simulink model "test_model_desktop_realtime"  (R2020b)
settings: Solver=FixedStepDiscrete  StartTime=0.0  StopTime=2  FixedStep=Ts  RelTol=1e-3
libraries: sldrtlib x1, simulink x1
settings Model: SimulationMode=external  ExtModeTrigDuration=100000  Creator=umbe  LastModifiedBy=irong
settings RTWCC: Description=Simulink Desktop Real-Time  SystemTargetFile=sldrt.tlc  TemplateMakefile=sldrt.tmf  RTWCompilerOptimization=on
settings CodeAppCC: MaxIdLength=95
settings SimulinkDesktopRealTimeCC: TargetPreCompLibLocation=D:\MATLAB\R2020b\toolbox\sldrt\lib\win64

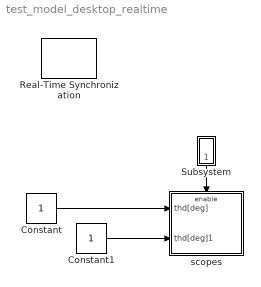
== system test_model_desktop_realtime ==
  Constant : Constant
  Constant1 : Constant
  Real-Time Synchronization : sldrtlib/Real-Time Synchronization  SampleTime=0.1  MaxMissedTicks=10  ShowMissedTicks=off  YieldWhenWaiting=off
  Subsystem : Subsystem
  scopes : Subsystem
  wires:
  Subsystem/1(1.0 s) -> scopes/Enable
  Constant/1 -> scopes/1(thd[deg])
  Constant1/1 -> scopes/2(thd[deg]1)

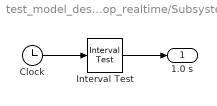
== system test_model_desktop_realtime/Subsystem ==
  Clock : Clock
  Interval Test : simulink/Logic and Bit Operations/Interval Test  IntervalClosedRight=on  uplimit=inf  IntervalClosedLeft=on  lowlimit=1  OutDataTypeStr=boolean
  1.0 s : Outport
  wires:
  Clock/1 -> Interval Test/1
  Interval Test/1 -> 1.0 s/1

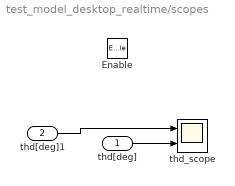
== system test_model_desktop_realtime/scopes ==
  thd[deg] : Inport
  thd[deg]1 : Inport  Port=2
  Enable : EnablePort
  thd_scope : Scope  NumInputPorts=2
  wires:
  thd[deg]/1 -> thd_scope/2
  thd[deg]1/1 -> thd_scope/1
